simulink model "callGAMS"  (R2021b)
settings: Solver=ode1  StartTime=0.0  StopTime=20  FixedStep=1e-4  RelTol=1e-3
model workspace (MAT data in the model file):
  firstOrder = 60
  g2Max = 0
  runTime = 4
undefined symbols (not defined in the file or in its folder): c0, c1, D11, Delta, fg, G2gen, G3gen, G5gen, G6gen, G7gen, Iovc, l0, l1, Newton, r0, r1, Raphson, Rtpu, S1non, S2non, S3non, S5non, S6non, S7non, sigbuilder_block, tonvsc, Ts, Vhv, Vmv, w_pll, wc1, wdc1, wpq1, wsw1, Xtpu
libraries: simulink_extras x122, simulink x73, spsFirstOrderFilterLib x72, spsGroundLib x61, spsCurrentMeasurementLib x33, spsVoltageMeasurementLib x33, eeTransforms x24, spsabctoAlphaBetaZeroLib x12, spsControlledVoltageSourceLib x12, spsControlledCurrentSourceLib x12, spsPower3phPhasorLib x11, spsLoadFlowBusLib x9
(part 16 of 16)

== system callGAMS/sm_computation/G6/VSC v2/VSC Control/Control loops/SW, EMT AVG, Phasor Quasi-EMT/Outer-loop/Subsystem2 ==
  note: Hold initial variable value for a given time
  In1 : Inport
  Constant : Constant  Value=x0
  Constant1 : Constant
  Integrator : Integrator
  Switch : Switch  Threshold=Td
  Out1 : Outport
  wires:
  Integrator/1 -> Switch/2
  In1/1 -> Switch/1
  Switch/1 -> Out1/1
  Constant/1 -> Switch/3
  Constant1/1 -> Integrator/1

== system callGAMS/sm_computation/G6/VSC v2/VSC Control/Control loops/SW, EMT AVG, Phasor Quasi-EMT/Outer-loop/Subsystem3 ==
  note: Hold initial variable value for a given time
  In1 : Inport
  Constant : Constant  Value=x0
  Constant1 : Constant
  Integrator : Integrator
  Switch : Switch  Threshold=Td
  Out1 : Outport
  wires:
  Integrator/1 -> Switch/2
  In1/1 -> Switch/1
  Switch/1 -> Out1/1
  Constant/1 -> Switch/3
  Constant1/1 -> Integrator/1

== system callGAMS/sm_computation/G6/VSC v2/VSC Control/Measurements/EMT/PLL aligned with positive-sequence/Phase-sequence separation ==
  note: Phase-sequence separation based on
      | Delayed Signal Cancellation (DSC) method
  abc : Inport
  Theta : Inport  Port=2
  Complex to Real-Imag1 : ComplexToRealImag
  Complex to Real-Imag2 : ComplexToRealImag
  Complex to Real-Imag3 : ComplexToRealImag
  Constant : Constant  Value=negseq_en
  Demux3 : Demux  Outputs=3
  Exp2 : Math  SignedPower=on  OutputSignalType=complex  SaturateOnIntegerOverflow=on
  Exp3 : Math  SignedPower=on  OutputSignalType=complex  SaturateOnIntegerOverflow=on
  Gain1 : Gain  Gain=1/2
  Gain4 : Gain  Gain=-1i
  Gain5 : Gain  Gain=1i
  Gain6 : Gain  Gain=1/2
  Gain7 : Gain  Gain=1i
  NOT : Logic  Operator=NOT  IconShape=distinctive  AllPortsSameDT=off  OutDataTypeStr=boolean
  Product3 : Product
  Product4 : Product
  Real-Imag to Complex : RealImagToComplex
  Real-Imag to Complex1 : RealImagToComplex
  Sum1 : Sum  Inputs=|++
  Sum2 : Sum  Inputs=-+|
  Switch : Switch  Criteria=u2 ~= 0
  Terminator3 : Terminator
  Transport Delay2 : TransportDelay  DelayTime=1/4*(1/fg)  BufferSize=1024*4
  Transport Delay3 : TransportDelay  DelayTime=1/4*(1/fg)  BufferSize=1024*4
  abc to Alpha-Beta-Zero : spsabctoAlphaBetaZeroLib/abc to Alpha-Beta-Zero
      settings: SourceProductBaseCode=PS
  q+ : Outport
  d+ : Outport  Port=2
  q- : Outport  Port=3
  d- : Outport  Port=4
  wires:
  NOT/1 -> Switch/2
  Constant/1 -> NOT/1
  Switch/1 -> Product3/1
  Gain6/1 -> Switch/3
  Sum2/1 -> Gain1/1
  Transport Delay2/1 -> Real-Imag to Complex1/1
  Demux3/1 -> Real-Imag to Complex/1
  Complex to Real-Imag1/2 -> Transport Delay3/1
  Gain1/1 -> Product4/2
  Real-Imag to Complex/1 -> Complex to Real-Imag1/1, Sum2/2, Sum1/1, Switch/1
  Complex to Real-Imag3/1 -> d-/1
  Real-Imag to Complex1/1 -> Gain5/1
  Complex to Real-Imag1/1 -> Transport Delay2/1
  Transport Delay3/1 -> Real-Imag to Complex1/2
  Demux3/2 -> Real-Imag to Complex/2
  Product3/1 -> Complex to Real-Imag2/1
  Product4/1 -> Complex to Real-Imag3/1
  abc to Alpha-Beta-Zero/1 -> Demux3/1
  abc/1 -> abc to Alpha-Beta-Zero/1
  Exp3/1 -> Product4/1
  Complex to Real-Imag3/2 -> q-/1
  Complex to Real-Imag2/2 -> q+/1
  Demux3/3 -> Terminator3/1
  Sum1/1 -> Gain6/1
  Gain5/1 -> Sum2/1, Sum1/2
  Exp2/1 -> Product3/2
  Gain4/1 -> Exp2/1
  Theta/1 -> Gain4/1, Gain7/1
  Gain7/1 -> Exp3/1
  Complex to Real-Imag2/1 -> d+/1

== system callGAMS/sm_computation/G6/VSC v2/VSC Control/Measurements/EMT/PLL aligned with positive-sequence/Subsystem ==
  note: PI controller with reset port and initial conditions restored after reset or after maximum/minimum values are reached
  in : Inport
  Reset : Inport  Port=2
  Compare To Constant2 : simulink/Logic and Bit Operations/Compare To Constant  relop=~=  const=0  OutDataTypeStr=boolean
  Constant2 : Constant  Value=2*pi*fg
  Gain : Gain  Gain=kp_pll
  Gain1 : Gain  Gain=kp_pll/tau_pll
  Integrator Limited : Integrator  ExternalReset=level  InitialCondition=2*pi*fg  UpperSaturationLimit=10.1*2*pi*fg  LowerSaturationLimit=0.09*2*pi*fg  ShowSaturationPort=on
  Memory1 : Memory
  NOT : Logic  Operator=NOT  IconShape=distinctive  AllPortsSameDT=off  OutDataTypeStr=boolean
  OR2 : Logic  Operator=OR  IconShape=distinctive  AllPortsSameDT=off  OutDataTypeStr=boolean
  Product : Product
  Sum : Sum
  Switch1 : Switch
  w : Outport
  wires:
  Switch1/1 -> w/1
  Product/1 -> Gain1/1, Gain/1
  Gain1/1 -> Integrator Limited/1
  Integrator Limited/2 -> Compare To Constant2/1, Switch1/2
  Compare To Constant2/1 -> Memory1/1
  OR2/1 -> Integrator Limited/2, NOT/1
  Constant2/1 -> Switch1/3
  Memory1/1 -> OR2/1
  Reset/1 -> OR2/2
  Gain/1 -> Sum/1
  Integrator Limited/1 -> Sum/2
  Sum/1 -> Switch1/1
  in/1 -> Product/1
  NOT/1 -> Product/2

== matlab function callGAMS/sc_user_interface/Real Time Redispatch Fn/MATLAB Function ==
  data: g2 output; g3 output; g5 output; g6 output; g2Reg output; g3Reg output; g5Reg output; g6Reg output; tsoComm input; totalGen output; pGenRT input; pPrev input; pExpected input
function [g2,g3,g5,g6,g2Reg,g3Reg,g5Reg,g6Reg,totalGen] = fcn(tsoComm,pGenRT,pPrev,pExpected)

    % Setup instruction to call GAMS

    filename = 'Redispatch_scenario1.xlsx';
    coder.extrinsic('callRtm')    

%     d = datetime;            % get current datetime
%     hStart = d.Hour;         % get the hour
%     tStart = d.Minute;       % get the minute

    hStart = 16;              % set the hour
    tStart = 1 ;              % set the minute

    timeD = 1;


    % Initialize active power set points    
    a = zeros(timeD,1);
    g2 = a;
    g3 = a;
    g5 = a;
    g6 = a;

    g2Reg = a;
    g3Reg = a;
    g5Reg = a;
    g6Reg = a;

    t    = zeros(60,1);
    pGen = {t,t,t,t};
    pReg = {t,t,t,t};

    mul = 1e6;
    megaWatt = 1e6;


    % Run GAMS file to get real-time updated set points
   
    [pGen,pReg,obj,~] = callRtm(tsoComm,hStart,tStart,pExpected,pGenRT,pPrev,filename);

    g2 = pGen{1,1}(1)*megaWatt ;
    g3 = pGen{1,2}(1)*megaWatt ;
    g5 = pGen{1,3}(1)*megaWatt ;
    g6 = pGen{1,4}(1)*megaWatt ;

    g2Reg = pReg{1,1}(1)*mul ;
    g3Reg = pReg{1,2}(1)*mul ;
    g5Reg = pReg{1,3}(1)*mul ;
    g6Reg = pReg{1,4}(1)*mul ;

    totalGen = ( g2   (1,1) + g3   (1,1) + g5   (1,1) + g6   (1,1) + ...
                 g2Reg(1,1) + g3Reg(1,1) + g5Reg(1,1) + g6Reg(1,1) );

    objective = obj ;

end
